simulink model "steering_pad_test_dual_no_tr"  (R2024b)
settings: Solver=VariableStepAuto  StartTime=0.0  StopTime=30  FixedStep=0.001  RelTol=1e-3
undefined symbols (not defined in the file): car
libraries: vehdynlibsteering x1, slpidlib x1, autolibshared x1
settings Model: Creator=Carlo  LastModifiedBy=giust

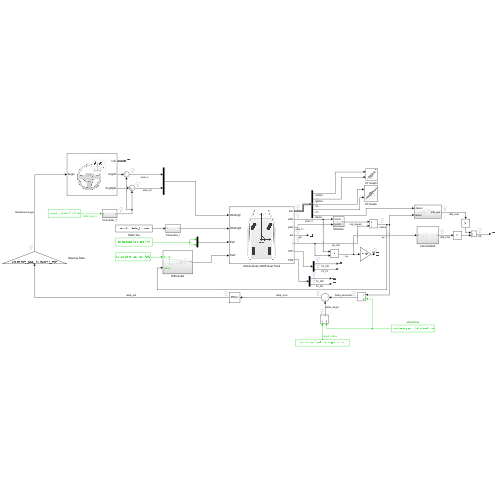
[thumbnail: Simulink's stored preview of the top-level diagram]
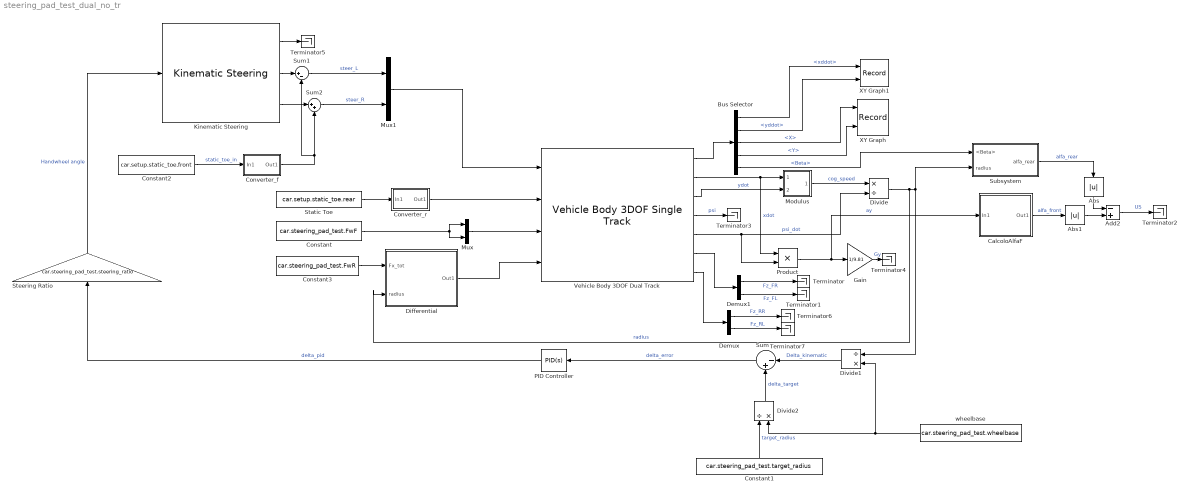
== system steering_pad_test_dual_no_tr ==
  Abs : Abs  SaturateOnIntegerOverflow=off
  Abs1 : Abs  SaturateOnIntegerOverflow=off
  Add2 : Sum  Inputs=-+
  Bus Selector : BusSelector  OutputSignals=BdyFrm.Cg.Acc.xddot,BdyFrm.Cg.Acc.yddot,InertFrm.Cg.Disp.X,InertFrm.Cg.Disp.Y,BdyFrm.Geom.Ang.Beta
  CalcoloAlfaF : Subsystem
  Constant : Constant  Value=car.steering_pad_test.FwF
  Constant1 : Constant  Value=car.steering_pad_test.target_radius
  Constant2 : Constant  Value=car.setup.static_toe.front
  Constant3 : Constant  Value=car.steering_pad_test.FwR
  Converter_f : Subsystem
  Converter_r : Subsystem
  Demux : Demux  Outputs=2
  Demux1 : Demux  Outputs=2
  Differential : Subsystem
  Divide : Product  Inputs=*/
  Divide1 : Product  Inputs=/*
  Divide2 : Product  Inputs=/*
  Gain : Gain  Gain=1/9.81
  Kinematic Steering : vehdynlibsteering/Kinematic Steering  StrgType=Ackerman  StrgRatioType=Constant  Loc=Front  NrmlFctr=car.kinematic_steering.NrmlFctr  TrckWdth=car.kinematic_steering.TrckWdth  WhlBase=car.kinematic_steering.WhlBase  Db=car.kinematic_steering.Db  StrgRng=car.kinematic_steering.StrgRng  StrgAngBpts="[-6.2832   -5.0265   -3.7699   -2.5133   -1.2566         0    1.2566    2.5133    3.7699    5.0265    6.2832]"  StrgRatioTbl=|  StrgRatio=car.kinematic_steering.StrgRatio  PctAckIn=off  PctAck=car.kinematic_steering.PctAck  PctAckTbl=ones(1,11)*100  StrgArmLngth=0.1  RckCsLngth=0.5  TieRodLngth=0.248  D=0.2  PnnRadius=0.00085818  PnnRadiusTbl="[0.0055    0.0055    0.0056    0.0057    0.0058    0.0057    0.0057    0.0057    0.0056    0.0055    0.0055]"  RodLngth=0.1  ParaArmLngth=0.9  aMode=2
      | [13.5000   13.3750   13.2500   13.1250   13.0000   13.0000   13.0000   13.1250   13.2500   13.3750   13.5000
      | ]
  Modulus : Subsystem
  Mux : Mux  Inputs=2
  Mux1 : Mux  Inputs=2
  PID Controller : slpidlib/PID Controller  Controller=PID  Form=Parallel  TimeDomain=Continuous-time  UseExternalTs=off  SampleTime=-1  IntegratorMethod=Forward Euler  FilterMethod=Forward Euler  ControllerParametersSource=internal  P=car.steering_pad_test.PID.P  I=car.steering_pad_test.PID.I  UseKiTs=off  D=car.steering_pad_test.PID.D  UseExternalDerivativeSource=off  N=car.steering_pad_test.PID.N  UseFilter=on  TunerSelectOption=Transfer Function Based (PID Tuner App)  InitialConditionSource=internal  InitialConditionForIntegrator=0  InitialConditionForFilter=0  DifferentiatorICPrevScaledInput=0  ExternalReset=none  TrackingMode=off  Kt=1  LimitOutput=off  SatLimitsSource=internal  UpperSaturationLimit=inf  LowerSaturationLimit=-inf  LinearizeAsGain=on  AntiWindupMode=none  Kb=1  LimitIntegrator=off  UpperIntegratorSaturationLimit=inf  LowerIntegratorSaturationLimit=-inf  POutMin=[]  POutMax=[]  IOutMin=[]  IOutMax=[]  DOutMin=[]  DOutMax=[]  NOutMin=[]  NOutMax=[]  SumOutMin=[]  SumOutMax=[]  SaturationOutMin=[]  SaturationOutMax=[]  PParamMin=[]  PParamMax=[]  IParamMin=[]  IParamMax=[]  DParamMin=[]  DParamMax=[]  NParamMin=[]  NParamMax=[]  KbParamMin=[]  KbParamMax=[]  KtParamMin=[]  KtParamMax=[]  KbOutMin=[]  KbOutMax=[]  KtOutMin=[]  KtOutMax=[]  IntegratorOutMin=[]  IntegratorOutMax=[]  FilterOutMin=[]  FilterOutMax=[]  SumI1OutMin=[]  SumI1OutMax=[]  SumI2OutMin=[]  SumI2OutMax=[]  SumI3OutMin=[]  SumI3OutMax=[]  SumI4OutMin=[]  SumI4OutMax=[]  SumDOutMin=[]  SumDOutMax=[]  DifferentiatorOutMin=[]  DifferentiatorOutMax=[]  FilterDiffOutCoefMin=[]  FilterDiffOutCoefMax=[]  ReciprocalOutMin=[]  ReciprocalOutMax=[]  SumDenOutMin=[]  SumDenOutMax=[]  SumNumOutMin=[]  SumNumOutMax=[]  DivideOutMin=[]  DivideOutMax=[]  UdiffTsProdOutMin=[]  UdiffTsProdOutMax=[]  NTsProdOutMin=[]  NTsProdOutMax=[]  UintegralTsProdOutMin=[]  UintegralTsProdOutMax=[]  UngainTsProdOutMin=[]  UngainTsProdOutMax=[]  ClampingZeroOutDataTypeStr=Inherit: Inherit via back propagation  ClampingZeroOutMin=[]  ClampingZeroOutMax=[]  FilterDenConstantOutDataTypeStr=Inherit: Inherit via back propagation  FilterDenConstantOutMin=[]  FilterDenConstantOutMax=[]  PCopyOutDataTypeStr=Inherit: Inherit via back propagation  PCopyOutMin=[]  PCopyOutMax=[]  NCopyOutDataTypeStr=Inherit: Inherit via back propagation  NCopyOutMin=[]  NCopyOutMax=[]  IntegratorContinuousStateAttributes=''  IntegratorStateMustResolveToSignalObject=off  IntegratorRTWStateStorageClass=Auto  FilterContinuousStateAttributes=''  FilterStateMustResolveToSignalObject=off  FilterRTWStateStorageClass=Auto  ParallelPVariant=InternalParameters  IdealPVariant=Disabled  IVariant=InternalParameters  DVariant=InternalParameters  IntegratorVariant=Continuous  SatVariant=Disabled  AWVariant=Passthrough  PCopyVariant=Disabled  TRVariant=Disabled  FdbkBlocksVariant=Forward  IdealPFdbkVariant=Disabled  SatFdbkVariant=Disabled  DerivativeFilterVariant=ContFilter  NVariant=InternalParameters  NCopyVariant=Disabled  FilterICVariant=InternalICsFilter  IntegratorICVariant=InternalICs  ExternalResetVariant=Disabled  TRSumVariant=Passthrough  SumFdbkVariant=Disabled  SumVariant=Sum_PID  TsampFilterVariant=InternalTs  TsampNgainVariant=Passthrough  TsampIntegralVariant=Disabled_SignalSpec  ExternalSaturationOutDataTypeStr=Inherit: Same as second input  DerivativeSourceVariant=ErrorSignal  PreIntVariant=InternalPreInt
  Product : Product
  Static Toe : Constant  Value=car.setup.static_toe.rear
  Steering Ratio : Gain  Gain=car.steering_pad_test.steering_ratio
  Subsystem : Subsystem
  Sum : Sum  Inputs=|-+
  Sum1 : Sum  Inputs=|+-
  Sum2 : Sum  Inputs=|++
  Terminator{,1..7} (8 alike) : Terminator
  Vehicle Body 3DOF Dual Track : autolibshared/Vehicle Body 3DOF Single Track  trackMode=Dual  inputMode=External longitudinal forces  frontSteerMode=on  rearSteerMode=on  windMode=off  muMode=off  extFMode=off  extMMode=off  htchFMode=off  htchMMode=off  extXo=off  extpsio=off  extxdoto=off  extro=off  extYo=off  extTamb=off  extydoto=off  aMode=2  NF=car.lateralbody.NF  NR=car.lateralbody.NR  m=car.lateralbody.m  a=car.lateralbody.a  b=car.lateralbody.b  h=car.lateralbody.h  dh=1  hh=0.2  X_o=car.lateralbody.X_o  xdot_o=car.lateralbody.xdot_o  CalphaMode=off  sigmaMode=on  d=car.lateralbody.d  hl=0  w=car.lateral.body.w  Cy_f=car.lateralbody.Cy_f  Cy_r=car.lateralbody.Cy_r  sigma_f=car.lateralbody.sigma_f  sigma_r=car.lateralbody.sigma_r  alpha_f_brk=[-.1 .1]  Cy_f_data=[-9e3 9e3]  alpha_r_brk=[-.1 .1]  Cy_r_data=[-9e3 9e3]  Y_o=car.lateralbody.Y_o  ydot_o=car.lateralbody.ydot_o  Izz=car.lateralbody.Izz  psi_o=car.lateralbody.psi_o  r_o=car.lateralbody.r_o  Af=car.lateralbody.Af  Cd=car.lateralbody.Cd  Cl=car.lateralbody.Cl  Cpm=car.lateralbody.Cpm  beta_w=car.lateralbody.beta_w  Cs=car.lateralbody.Cs  Cym=car.lateralbody.Cym  Pabs=car.lateralbody.Pabs  Tair=car.lateralbody.Tair  g=car.lateralbody.g  mu=car.lateralbody.mu  xdot_tol=car.lateralbody.xdot_tol  Fznom=car.lateralbody.Fznom  Fxtire_sat=7e4  Fytire_sat=7e4  longOff=car.lateralbody.longOff  latOff=car.lateralbody.latOff  vertOff=car.lateralbody.vertOff  wrapAng=off
      settings: LibrarySourceBlock=vehdynlibeom/Vehicle Body 3DOF Dual Track
  XY Graph : Record  FileSettingsInternal="{\"entries\":[{\"content\":{\"excelSettings\":{\"content\":{},\"type\":\"Streamout.ExcelSettings\"}},\"type\":\"Streamout.FileSettingStorage\",\"uuid\":\"\"}],\"packageUris\":[\"http:\\/\\/schema.mathworks.com\\/mf0\\/streamout_blocks\\/R2020a\"],\"version\":\"1.0\"}"  Layout=[1 1]  SignalsInternal="{\"entries\":[{\"content\":{\"signals\":[{\"content\":{\"blockPath\":[],\"dimensions\":[1],\"domain\":\"\",\"lineColor\":\"#a2142f\",\"plots\":[ 1 ],\"port\":1,\"sid\":[\"\"],\"signalID\":1,\"signalName\":\"<X>\"},\"type\":\"RecordBlkView.Signal\",\"uuid\":\"\"},{\"content\":{\"blockPath\":[],\"dimensions\":[1],\"domain\":\"\",\"lineColor\":\"#139fff\",\"plots\":[ 1 ],\"port\":2,\"sid\":[\"\"],\"signalID\":2,\"signalName\":\"<Y>\"},\"type\":\"RecordBlkView.Signal\",\"uuid\":\"\"}]},\"type\":\"RecordBlkView.InputSignals\",\"uuid\":\"\"}],\"packageUris\":[\"http:\\/\\/schema.mathworks.com\\/mf0\\/streamout_blocks\\/R2020a\"],\"version\":\"1.0\"}"  VisualizationBindings="{\"xyplotplugin\":{\"info\":[{\"series\":[{\"bindingParametersList\":[{\"parameter\":\"X-Axis\",\"signalID\":1,\"signalName\":\"<X>\"},{\"parameter\":\"Y-Axis\",\"signalID\":2,\"signalName\":\"<Y>\"}],\"seriesID\":0}],\"subplotID\":1}]}}"  CompatibilityTag=XY
  XY Graph1 : Record  FileSettingsInternal="{\"entries\":[{\"content\":{\"excelSettings\":{\"content\":{},\"type\":\"Streamout.ExcelSettings\"}},\"type\":\"Streamout.FileSettingStorage\",\"uuid\":\"\"}],\"packageUris\":[\"http:\\/\\/schema.mathworks.com\\/mf0\\/streamout_blocks\\/R2020a\"],\"version\":\"1.0\"}"  Layout=[1 1]  SignalsInternal="{\"entries\":[{\"content\":{\"signals\":[{\"content\":{\"blockPath\":[],\"dimensions\":[1],\"domain\":\"\",\"lineColor\":\"#a2142f\",\"plots\":[ 1 ],\"port\":1,\"sid\":[\"\"],\"signalID\":1,\"signalName\":\"<xddot>\"},\"type\":\"RecordBlkView.Signal\",\"uuid\":\"\"},{\"content\":{\"blockPath\":[],\"dimensions\":[1],\"domain\":\"\",\"lineColor\":\"#139fff\",\"plots\":[ 1 ],\"port\":2,\"sid\":[\"\"],\"signalID\":2,\"signalName\":\"<yddot>\"},\"type\":\"RecordBlkView.Signal\",\"uuid\":\"\"}]},\"type\":\"RecordBlkView.InputSignals\",\"uuid\":\"\"}],\"packageUris\":[\"http:\\/\\/schema.mathworks.com\\/mf0\\/streamout_blocks\\/R2020a\"],\"version\":\"1.0\"}"  VisualizationBindings="{\"xyplotplugin\":{\"info\":[{\"series\":[{\"bindingParametersList\":[{\"parameter\":\"X-Axis\",\"signalID\":1,\"signalName\":\"<xddot>\"},{\"parameter\":\"Y-Axis\",\"signalID\":2,\"signalName\":\"<yddot>\"}],\"seriesID\":0}],\"subplotID\":1}]}}"  CompatibilityTag=XY
  wheelbase : Constant  Value=car.steering_pad_test.wheelbase
  wires:
  Vehicle Body 3DOF Dual Track/7 -> Demux/1
  Vehicle Body 3DOF Dual Track/6 -> Demux1/1
  Vehicle Body 3DOF Dual Track/5 -> Product/2, Divide/2  "psi_dot"
  Vehicle Body 3DOF Dual Track/4 -> Terminator3/1  "psi"
  Vehicle Body 3DOF Dual Track/1 -> Bus Selector/1
  Bus Selector/3 -> XY Graph/1  "<X>"
  Bus Selector/4 -> XY Graph/2  "<Y>"
  Vehicle Body 3DOF Dual Track/2 -> Product/1, Modulus/1(<xdot>)  "xdot"
  Vehicle Body 3DOF Dual Track/3 -> Modulus/2(<ydot>)  "ydot"
  Modulus/1(Out1) -> Divide/1  "cog_speed"
  Divide/1 -> Differential/2(radius), Subsystem/2(radius), Divide1/1  "radius"
  Bus Selector/5 -> Subsystem/1(<Beta>)  "<Beta>"
  Product/1 -> CalcoloAlfaF/1(In1), Gain/1  "ay"
  Divide1/1 -> Sum/1  "Delta_kinematic"
  Steering Ratio/1 -> Kinematic Steering/1  "Handwheel angle"
  Kinematic Steering/3 -> Sum2/1
  Kinematic Steering/2 -> Sum1/1
  Mux1/1 -> Vehicle Body 3DOF Dual Track/1
  Kinematic Steering/1 -> Terminator5/1
  wheelbase/1 -> Divide1/2, Divide2/2
  Divide2/1 -> Sum/2  "delta_target"
  Sum/1 -> PID Controller/1  "delta_error"
  PID Controller/1 -> Steering Ratio/1  "delta_pid"
  Sum1/1 -> Mux1/1  "steer_L"
  Sum2/1 -> Mux1/2  "steer_R"
  Constant2/1 -> Converter_f/1(In1)  "static_toe_in"
  Mux/1 -> Vehicle Body 3DOF Dual Track/3
  Constant/1 -> Mux/2, Mux/1
  Demux1/1 -> Terminator/1  "Fz_FR"
  Demux1/2 -> Terminator1/1  "Fz_FL"
  Demux/1 -> Terminator6/1  "Fz_RR"
  Demux/2 -> Terminator7/1  "Fz_RL"
  Subsystem/1(alfa_rear) -> Abs/1  "alfa_rear"
  Gain/1 -> Terminator4/1  "Gy"
  CalcoloAlfaF/1(Out1) -> Abs1/1  "alfa_front"
  Add2/1 -> Terminator2/1  "US"
  Abs/1 -> Add2/1
  Abs1/1 -> Add2/2
  Differential/1(Out1) -> Vehicle Body 3DOF Dual Track/4
  Constant3/1 -> Differential/1(Fx_tot)
  Constant1/1 -> Divide2/1  "target_radius"
  Static Toe/1 -> Converter_r/1(In1)
  Converter_r/1(Out1) -> Vehicle Body 3DOF Dual Track/2
  Converter_f/1(Out1) -> Sum1/2, Sum2/2
  Bus Selector/1 -> XY Graph1/1  "<xddot>"
  Bus Selector/2 -> XY Graph1/2  "<yddot>"

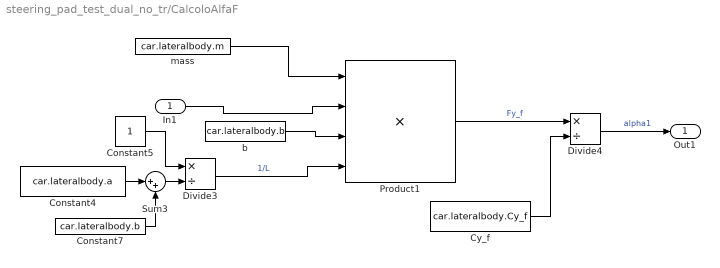
== system steering_pad_test_dual_no_tr/CalcoloAlfaF ==
  In1 : Inport
  Constant4 : Constant  Value=car.lateralbody.a
  Constant5 : Constant
  Constant7 : Constant  Value=car.lateralbody.b
  Cy_f : Constant  Value=car.lateralbody.Cy_f
  Divide3 : Product  Inputs=*/
  Divide4 : Product  Inputs=*/
  Product1 : Product  Inputs=4
  Sum3 : Sum  Inputs=|++
  b : Constant  Value=car.lateralbody.b
  mass : Constant  Value=car.lateralbody.m
  Out1 : Outport
  wires:
  mass/1 -> Product1/1
  Divide3/1 -> Product1/4  "1/L"
  Sum3/1 -> Divide3/2
  b/1 -> Product1/3
  Constant4/1 -> Sum3/1
  Constant5/1 -> Divide3/1
  Divide4/1 -> Out1/1  "alpha1"
  Constant7/1 -> Sum3/2
  Product1/1 -> Divide4/1  "Fy_f"
  Cy_f/1 -> Divide4/2
  In1/1 -> Product1/2

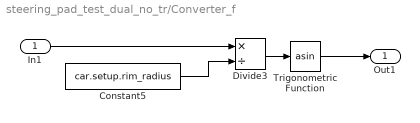
== system steering_pad_test_dual_no_tr/Converter_f ==
  In1 : Inport
  Constant5 : Constant  Value=car.setup.rim_radius  VectorParams1D=off
  Divide3 : Product  Inputs=*/
  Trigonometric Function : Trigonometry  Operator=asin
  Out1 : Outport
  wires:
  In1/1 -> Divide3/1
  Divide3/1 -> Trigonometric Function/1
  Trigonometric Function/1 -> Out1/1
  Constant5/1 -> Divide3/2

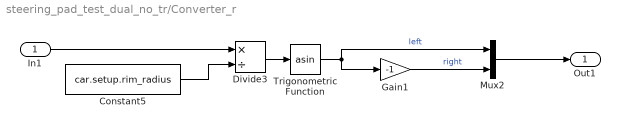
== system steering_pad_test_dual_no_tr/Converter_r ==
  In1 : Inport
  Constant5 : Constant  Value=car.setup.rim_radius  VectorParams1D=off
  Divide3 : Product  Inputs=*/
  Gain1 : Gain  Gain=-1
  Mux2 : Mux  Inputs=2
  Trigonometric Function : Trigonometry  Operator=asin
  Out1 : Outport
  wires:
  In1/1 -> Divide3/1
  Gain1/1 -> Mux2/2  "right"
  Divide3/1 -> Trigonometric Function/1
  Trigonometric Function/1 -> Mux2/1, Gain1/1  "left"
  Constant5/1 -> Divide3/2
  Mux2/1 -> Out1/1

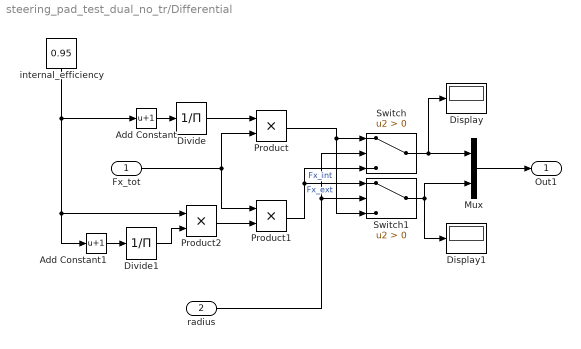
== system steering_pad_test_dual_no_tr/Differential ==
  Fx_tot : Inport
  radius : Inport  Port=2
  Add Constant : Bias  Bias=1  SaturateOnIntegerOverflow=off
  Add Constant1 : Bias  Bias=1  SaturateOnIntegerOverflow=off
  Display : Display
  Display1 : Display
  Divide : Product  Inputs=/
  Divide1 : Product  Inputs=/
  Mux : Mux  Inputs=2
  Product : Product
  Product1 : Product
  Product2 : Product
  Switch : Switch  Criteria=u2 > Threshold  SaturateOnIntegerOverflow=off  InputSameDT=off
  Switch1 : Switch  Criteria=u2 > Threshold  SaturateOnIntegerOverflow=off  InputSameDT=off
  internal_efficiency : Constant  Value=0.95
  Out1 : Outport
  wires:
  Mux/1 -> Out1/1
  Fx_tot/1 -> Product1/1, Product/2
  Add Constant/1 -> Divide/1
  internal_efficiency/1 -> Product2/1, Add Constant1/1, Add Constant/1
  Divide/1 -> Product/1
  Add Constant1/1 -> Divide1/1
  Divide1/1 -> Product2/2
  Product2/1 -> Product1/2
  Product/1 -> Switch/1, Switch1/3  "Fx_int"
  radius/1 -> Switch1/2, Switch/2
  Switch/1 -> Display/1, Mux/1
  Product1/1 -> Switch1/1, Switch/3  "Fx_ext"
  Switch1/1 -> Display1/1, Mux/2

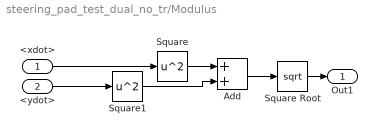
== system steering_pad_test_dual_no_tr/Modulus ==
  <xdot> : Inport
  <ydot> : Inport  Port=2
  Add : Sum
  Square : Math  Operator=square
  Square Root : Sqrt
  Square1 : Math  Operator=square
  Out1 : Outport
  wires:
  Add/1 -> Square Root/1
  Square/1 -> Add/1
  Square1/1 -> Add/2
  Square Root/1 -> Out1/1
  <ydot>/1 -> Square1/1
  <xdot>/1 -> Square/1

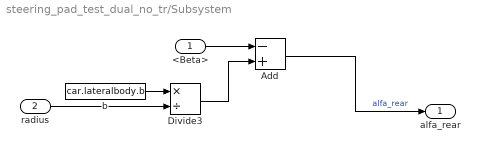
== system steering_pad_test_dual_no_tr/Subsystem ==
  <Beta> : Inport
  radius : Inport  Port=2
  Add : Sum  Inputs=-+
  Divide3 : Product  Inputs=*/
  b : Constant  Value=car.lateralbody.b
  alfa_rear : Outport
  wires:
  radius/1 -> Divide3/2
  Add/1 -> alfa_rear/1  "alfa_rear"
  Divide3/1 -> Add/2
  b/1 -> Divide3/1
  <Beta>/1 -> Add/1
